simulink model "sampleModel1935"  (R2023a)
settings: Solver=VariableStepAuto  StartTime=0.0  StopTime=10.0  RelTol=1e-3
libraries: hdlsllib x5, simulink x3
settings Model: Creator=user1  LastModifiedBy=user1

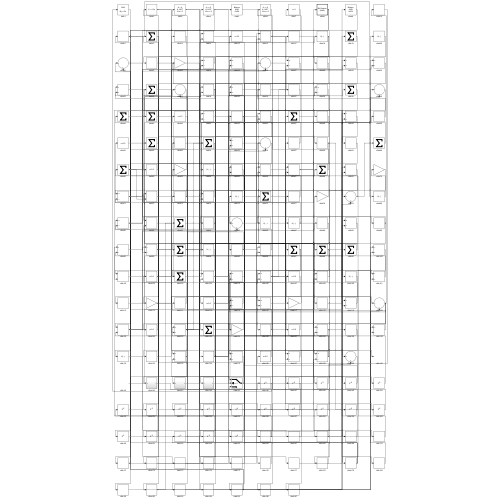
[thumbnail: Simulink's stored preview of the top-level diagram]
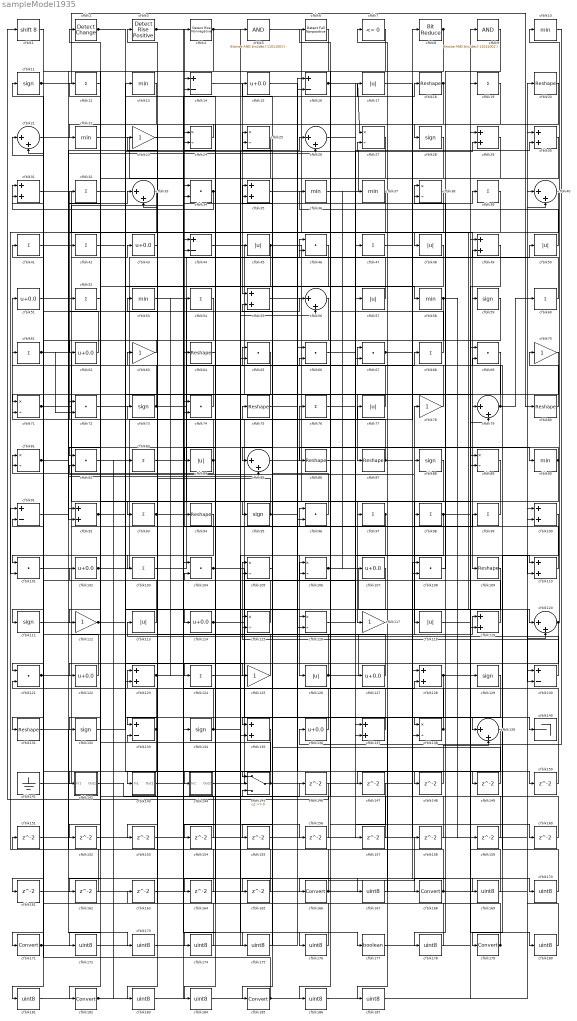
== system sampleModel1935 ==
  cfblk1 : ArithShift  BitShiftNumber=8
  cfblk{10,13,22,36..37,53,58,90} (8 alike) : MinMax
  cfblk{29..31,35,49,55,92,100,110,119,123,128,135,137} (14 alike) : Sum
  cfblk{34,46,65..67,69,72,74,82,96,101,104,108,121} (14 alike) : DotProduct  OutDataTypeStr=Inherit: Inherit via internal rule
  cfblk{15,43,51,62,102,107,114,122,127,136} (10 alike) : Bias  Bias=0.0  SaturateOnIntegerOverflow=off
  cfblk{12,19,32,39,41..42,47,52,54,60..61,68,76,83,93,97..99,103,124} (20 alike) : Sum  Inputs=+
  cfblk{24..25,27,38,71,81,89,105..106,115..116,138} (12 alike) : Product  Inputs=*/  RndMeth=Zero  SaturateOnIntegerOverflow=on
  cfblk{18,20,64,75,80,86..87,94,109,131} (10 alike) : Reshape
  cfblk{11,28,59,73,88,95,111,129,132,134} (10 alike) : Signum
  cfblk{23,63,70,78,112,117,125} (7 alike) : Gain
  cfblk{17,45,48,50,57,77,84,113,118,126} (10 alike) : Abs  SaturateOnIntegerOverflow=off
  cfblk{21,26,33,40,56,79,85,120,139} (9 alike) : Sum  Inputs=|++
  cfblk{14,16,44,91,130,133} (6 alike) : Sum  Inputs=+-
  cfblk140 : Terminator
  cfblk141 : Ground
  cfblk142 : Subsystem
      settings: LibrarySourceBlock=|
      | hdlsllib/Ports &
      | Subsystems/Subsystem
  cfblk143 : Subsystem
      settings: LibrarySourceBlock=|
      | hdlsllib/Ports &
      | Subsystems/Subsystem
  cfblk144 : Subsystem
      settings: LibrarySourceBlock=|
      | hdlsllib/Ports &
      | Subsystems/Subsystem
  cfblk145 : Switch  SaturateOnIntegerOverflow=off  InputSameDT=off
  cfblk{146..165} (20 alike) : Delay  SampleTime=1
  cfblk{166,168,171,179,182,185} (6 alike) : DataTypeConversion  SaturateOnIntegerOverflow=off  RndMeth=Floor
  cfblk{167,169..170,172..176,178,180..181,183..184,186..187} (15 alike) : DataTypeConversion  OutDataTypeStr=uint8  SaturateOnIntegerOverflow=off  RndMeth=Floor
  cfblk177 : DataTypeConversion  OutDataTypeStr=boolean  SaturateOnIntegerOverflow=off  RndMeth=Floor
  cfblk2 : simulink/Logic and Bit Operations/Detect Change  vinit=0  OutDataTypeStr=boolean
      settings: LibrarySourceBlock=|
      | hdlsllib/Logic and Bit
      | Operations/Detect
      | Change
  cfblk3 : hdlsllib/Logic and Bit Operations/Detect Rise Positive  vinit=0  OutDataTypeStr=boolean
  cfblk4 : hdlsllib/Logic and Bit Operations/Detect Rise Nonnegative  vinit=0  OutDataTypeStr=boolean
  cfblk5 : simulink/Logic and Bit Operations/Bitwise Operator  logicop=AND  UseBitMask=on  BitMask=bin2dec('11011001')  BitMaskRealWorld=Stored Integer
      settings: LibrarySourceBlock=|
      | hdlsllib/Logic and Bit
      | Operations/Bitwise
      | Operator
  cfblk6 : hdlsllib/Logic and Bit Operations/Detect Fall Nonpositive  vinit=0  OutDataTypeStr=boolean
  cfblk7 : hdlsllib/Logic and Bit Operations/Compare To Zero  relop=<=  OutDataTypeStr=boolean
  cfblk8 : hdlsllib/Logic and Bit Operations/Bit Reduce  mode=AND
  cfblk9 : simulink/Logic and Bit Operations/Bitwise Operator  logicop=AND  UseBitMask=on  BitMask=bin2dec('11011001')  BitMaskRealWorld=Stored Integer
      settings: LibrarySourceBlock=|
      | hdlsllib/Logic and Bit
      | Operations/Bitwise
      | Operator
  wires:
  cfblk111/1 -> cfblk43/1
  cfblk104/1 -> cfblk138/1, cfblk38/2
  cfblk39/1 -> cfblk109/1
  cfblk51/1 -> cfblk33/1
  cfblk57/1 -> cfblk4/1
  cfblk35/1 -> cfblk120/1
  cfblk93/1 -> cfblk68/1, cfblk156/1
  cfblk79/1 -> cfblk51/1, cfblk60/1
  cfblk69/1 -> cfblk168/1
  cfblk103/1 -> cfblk46/1
  cfblk144/1(Out1) -> cfblk8/1
  cfblk110/1 -> cfblk14/1
  cfblk141/1 -> cfblk34/1
  cfblk4/1 -> cfblk5/1, cfblk97/1, cfblk172/1
  cfblk80/1 -> cfblk70/1
  cfblk97/1 -> cfblk126/1, cfblk116/2
  cfblk130/1 -> cfblk113/1
  cfblk109/1 -> cfblk133/1
  cfblk68/1 -> cfblk44/1
  cfblk53/1 -> cfblk117/1
  cfblk5/1 -> cfblk59/1
  cfblk56/1 -> cfblk143/1(In1)
  cfblk86/1 -> cfblk137/1
  cfblk11/1 -> cfblk80/1, cfblk48/1
  cfblk41/1 -> cfblk34/2
  cfblk138/1 -> cfblk96/1, cfblk115/1
  cfblk25/1 -> cfblk44/2
  cfblk128/1 -> cfblk147/1, cfblk180/1
  cfblk108/1 -> cfblk38/1
  cfblk44/1 -> cfblk87/1
  cfblk24/1 -> cfblk22/1
  cfblk34/1 -> cfblk124/1, cfblk31/2
  cfblk102/1 -> cfblk77/1, cfblk27/2
  cfblk89/1 -> cfblk182/1
  cfblk21/1 -> cfblk90/1
  cfblk59/1 -> cfblk137/2
  cfblk126/1 -> cfblk78/1, cfblk55/2
  cfblk84/1 -> cfblk52/1, cfblk81/2
  cfblk62/1 -> cfblk41/1
  cfblk90/1 -> cfblk86/1, cfblk153/1
  cfblk120/1 -> cfblk10/1, cfblk122/1, cfblk115/2, cfblk145/2
  cfblk10/1 -> cfblk136/1
  cfblk46/1 -> cfblk144/1(In1)
  cfblk61/1 -> cfblk118/1, cfblk72/2, cfblk56/1
  cfblk76/1 -> cfblk110/1
  cfblk121/1 -> cfblk119/1, cfblk85/2, cfblk24/2
  cfblk32/1 -> cfblk58/1
  cfblk98/1 -> cfblk49/1, cfblk135/2
  cfblk73/1 -> cfblk30/1, cfblk32/1
  cfblk22/1 -> cfblk134/1
  cfblk132/1 -> cfblk99/1
  cfblk6/1 -> cfblk101/1
  cfblk7/1 -> cfblk166/1
  cfblk8/1 -> cfblk92/2, cfblk181/1
  cfblk40/1 -> cfblk185/1
  cfblk133/1 -> cfblk21/2, cfblk152/1
  cfblk63/1 -> cfblk62/1
  cfblk112/1 -> cfblk13/1, cfblk116/1
  cfblk55/1 -> cfblk129/1
  cfblk99/1 -> cfblk93/1
  cfblk87/1 -> cfblk61/1, cfblk110/2
  cfblk14/1 -> cfblk55/1
  cfblk71/1 -> cfblk127/1, cfblk26/1
  cfblk143/1(Out1) -> cfblk39/1
  cfblk1/1 -> cfblk71/1
  cfblk100/1 -> cfblk179/1
  cfblk29/1 -> cfblk142/1(In1)
  cfblk119/1 -> cfblk81/1
  cfblk13/1 -> cfblk132/1
  cfblk43/1 -> cfblk103/1
  cfblk127/1 -> cfblk105/1
  cfblk101/1 -> cfblk47/1
  cfblk134/1 -> cfblk123/1, cfblk29/2, cfblk56/2, cfblk176/1
  cfblk114/1 -> cfblk57/1, cfblk66/2
  cfblk18/1 -> cfblk28/1, cfblk183/1
  cfblk16/1 -> cfblk27/1, cfblk160/1
  cfblk115/1 -> cfblk24/1
  cfblk38/1 -> cfblk111/1
  cfblk106/1 -> cfblk130/2, cfblk37/1, cfblk107/1
  cfblk122/1 -> cfblk31/1
  cfblk118/1 -> cfblk50/1
  cfblk49/1 -> cfblk119/2
  cfblk72/1 -> cfblk20/1
  cfblk96/1 -> cfblk63/1
  cfblk88/1 -> cfblk114/1
  cfblk77/1 -> cfblk25/1
  cfblk95/1 -> cfblk16/1, cfblk23/1
  cfblk105/1 -> cfblk35/1
  cfblk52/1 -> cfblk12/1
  cfblk36/1 -> cfblk19/1
  cfblk92/1 -> cfblk139/1, cfblk17/1
  cfblk117/1 -> cfblk67/1
  cfblk3/1 -> cfblk98/1, cfblk170/1
  cfblk58/1 -> cfblk131/1, cfblk159/1
  cfblk124/1 -> cfblk106/1
  cfblk67/1 -> cfblk140/1, cfblk49/2
  cfblk116/1 -> cfblk67/2
  cfblk60/1 -> cfblk6/1
  cfblk136/1 -> cfblk104/2
  cfblk23/1 -> cfblk64/1
  cfblk75/1 -> cfblk16/2
  cfblk27/1 -> cfblk85/1
  cfblk45/1 -> cfblk128/1, cfblk82/1
  cfblk74/1 -> cfblk33/2
  cfblk48/1 -> cfblk95/1
  cfblk125/1 -> cfblk73/1
  cfblk91/1 -> cfblk88/1
  cfblk42/1 -> cfblk25/2
  cfblk28/1 -> cfblk135/1
  cfblk82/1 -> cfblk125/1
  cfblk107/1 -> cfblk123/2
  cfblk30/1 -> cfblk84/1
  cfblk85/1 -> cfblk76/1
  cfblk113/1 -> cfblk2/1
  cfblk94/1 -> cfblk171/1
  cfblk66/1 -> cfblk30/2
  cfblk81/1 -> cfblk42/1, cfblk26/2
  cfblk137/1 -> cfblk65/1
  cfblk123/1 -> cfblk128/2, cfblk53/1, cfblk18/1, cfblk54/1, cfblk177/1
  cfblk12/1 -> cfblk112/1
  cfblk50/1 -> cfblk36/1
  cfblk70/1 -> cfblk121/1
  cfblk145/1 -> cfblk108/2, cfblk72/1
  cfblk2/1 -> cfblk145/1, cfblk79/1
  cfblk33/1 -> cfblk101/2
  cfblk31/1 -> cfblk65/2
  cfblk78/1 -> cfblk11/1
  cfblk142/1(Out1) -> cfblk146/1
  cfblk146/1 -> cfblk1/1
  cfblk15/1 -> cfblk148/1
  cfblk148/1 -> cfblk139/2
  cfblk83/1 -> cfblk149/1
  cfblk149/1 -> cfblk105/2
  cfblk47/1 -> cfblk150/1
  cfblk150/1 -> cfblk74/1
  cfblk152/1 -> cfblk120/2
  cfblk153/1 -> cfblk104/1
  cfblk65/1 -> cfblk154/1
  cfblk154/1 -> cfblk133/2
  cfblk129/1 -> cfblk155/1
  cfblk155/1 -> cfblk138/2
  cfblk156/1 -> cfblk35/2
  cfblk26/1 -> cfblk157/1
  cfblk157/1 -> cfblk106/2
  cfblk158/1 -> cfblk108/1
  cfblk159/1 -> cfblk82/2
  cfblk160/1 -> cfblk46/2
  cfblk135/1 -> cfblk161/1
  cfblk161/1 -> cfblk130/1
  cfblk54/1 -> cfblk162/1
  cfblk162/1 -> cfblk92/1
  cfblk64/1 -> cfblk164/1
  cfblk164/1 -> cfblk91/1
  cfblk37/1 -> cfblk165/1
  cfblk165/1 -> cfblk71/2
  cfblk166/1 -> cfblk158/1, cfblk102/1
  cfblk131/1 -> cfblk167/1
  cfblk167/1 -> cfblk7/1
  cfblk168/1 -> cfblk79/2, cfblk75/1
  cfblk17/1 -> cfblk169/1
  cfblk169/1 -> cfblk69/1
  cfblk170/1 -> cfblk69/2
  cfblk171/1 -> cfblk21/1, cfblk45/1
  cfblk172/1 -> cfblk94/1
  cfblk151/1 -> cfblk173/1
  cfblk173/1 -> cfblk96/2
  cfblk20/1 -> cfblk174/1
  cfblk174/1 -> cfblk151/1
  cfblk163/1 -> cfblk175/1
  cfblk175/1 -> cfblk145/3
  cfblk176/1 -> cfblk163/1
  cfblk177/1 -> cfblk9/1
  cfblk9/1 -> cfblk178/1
  cfblk178/1 -> cfblk3/1
  cfblk179/1 -> cfblk14/2, cfblk66/1, cfblk15/1
  cfblk180/1 -> cfblk100/1
  cfblk181/1 -> cfblk100/2
  cfblk182/1 -> cfblk74/2, cfblk83/1
  cfblk183/1 -> cfblk89/1
  cfblk19/1 -> cfblk184/1
  cfblk184/1 -> cfblk89/2
  cfblk185/1 -> cfblk121/2, cfblk91/2, cfblk29/1
  cfblk147/1 -> cfblk186/1
  cfblk186/1 -> cfblk40/1
  cfblk139/1 -> cfblk187/1
  cfblk187/1 -> cfblk40/2

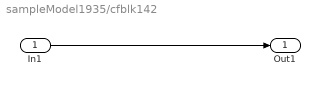
== system sampleModel1935/cfblk142 ==
  In1 : Inport
  Out1 : Outport
  wires:
  In1/1 -> Out1/1

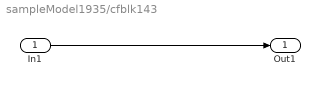
== system sampleModel1935/cfblk143 ==
  In1 : Inport
  Out1 : Outport
  wires:
  In1/1 -> Out1/1

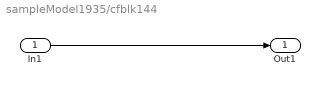
== system sampleModel1935/cfblk144 ==
  In1 : Inport
  Out1 : Outport
  wires:
  In1/1 -> Out1/1
